simulink model "path_following_PID_v2"  (R2022a)
settings: Solver=VariableStepAuto  StartTime=0.0  StopTime=10  RelTol=1e-3
values from neighbouring files (symbols this model uses):
  ref = [x_ref, y_ref]    [reference.m]
libraries: slpidlib x1
settings Model: Creator=andreagottardini  LastModifiedBy=andreagottardini

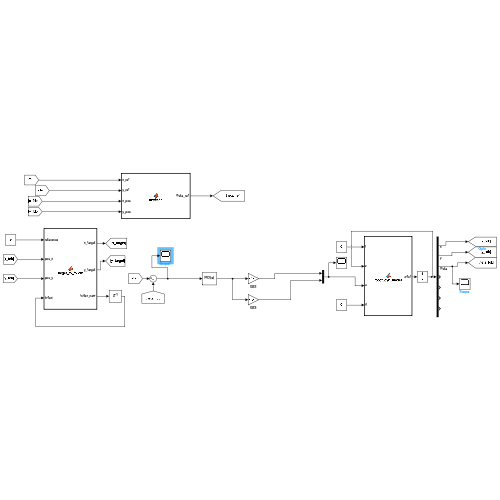
[thumbnail: Simulink's stored preview of the top-level diagram]
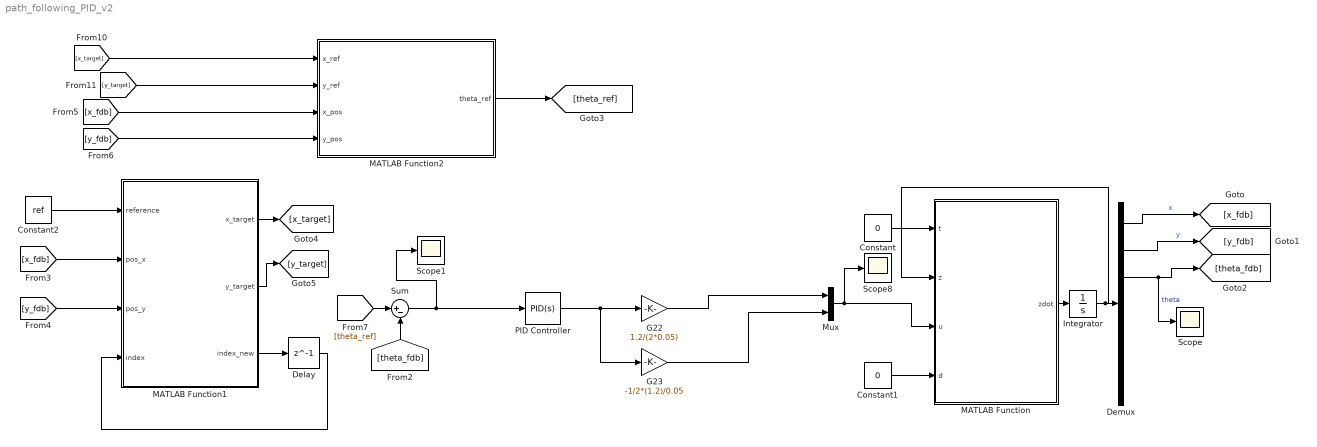
== system path_following_PID_v2 ==
  Constant : Constant  Value=0
  Constant1 : Constant  Value=0
  Constant2 : Constant  Value=ref
  Delay : Delay  DelayLength=1  InitialCondition=1
  Demux : Demux  Outputs=7
  G22 : Gain  Gain=1.2/(2*0.05)
  G23 : Gain  Gain=-1/2*(1.2)/0.05
  Integrator : Integrator  InitialCondition=[0;0;0;0;0;0;0]
  MATLAB Function : MATLAB Function  TreatAsAtomicUnit=on
  MATLAB Function1 : MATLAB Function  TreatAsAtomicUnit=on
  MATLAB Function2 : MATLAB Function  TreatAsAtomicUnit=on
  Mux : Mux  Inputs=2
  PID Controller : slpidlib/PID Controller  Controller=PID  Form=Parallel  TimeDomain=Continuous-time  UseExternalTs=off  SampleTime=-1  IntegratorMethod=Forward Euler  FilterMethod=Forward Euler  ControllerParametersSource=internal  P=0  I=1  UseKiTs=off  D=0  N=30  UseFilter=on  TunerSelectOption=Transfer Function Based (PID Tuner App)  InitialConditionSource=internal  InitialConditionForIntegrator=0  InitialConditionForFilter=0  DifferentiatorICPrevScaledInput=0  ExternalReset=none  TrackingMode=off  Kt=1  LimitOutput=off  SatLimitsSource=internal  UpperSaturationLimit=inf  LowerSaturationLimit=-inf  LinearizeAsGain=on  AntiWindupMode=none  Kb=1  POutMin=[]  POutMax=[]  IOutMin=[]  IOutMax=[]  DOutMin=[]  DOutMax=[]  NOutMin=[]  NOutMax=[]  SumOutMin=[]  SumOutMax=[]  SaturationOutMin=[]  SaturationOutMax=[]  PParamMin=[]  PParamMax=[]  IParamMin=[]  IParamMax=[]  DParamMin=[]  DParamMax=[]  NParamMin=[]  NParamMax=[]  KbParamMin=[]  KbParamMax=[]  KtParamMin=[]  KtParamMax=[]  KbOutMin=[]  KbOutMax=[]  KtOutMin=[]  KtOutMax=[]  IntegratorOutMin=[]  IntegratorOutMax=[]  FilterOutMin=[]  FilterOutMax=[]  SumI1OutMin=[]  SumI1OutMax=[]  SumI2OutMin=[]  SumI2OutMax=[]  SumI3OutMin=[]  SumI3OutMax=[]  SumI4OutMin=[]  SumI4OutMax=[]  SumDOutMin=[]  SumDOutMax=[]  DifferentiatorOutMin=[]  DifferentiatorOutMax=[]  FilterDiffOutCoefMin=[]  FilterDiffOutCoefMax=[]  ReciprocalOutMin=[]  ReciprocalOutMax=[]  SumDenOutMin=[]  SumDenOutMax=[]  SumNumOutMin=[]  SumNumOutMax=[]  DivideOutMin=[]  DivideOutMax=[]  UdiffTsProdOutMin=[]  UdiffTsProdOutMax=[]  NTsProdOutMin=[]  NTsProdOutMax=[]  UintegralTsProdOutMin=[]  UintegralTsProdOutMax=[]  UngainTsProdOutMin=[]  UngainTsProdOutMax=[]  IntegratorContinuousStateAttributes=''  IntegratorStateMustResolveToSignalObject=off  IntegratorRTWStateStorageClass=Auto  FilterContinuousStateAttributes=''  FilterStateMustResolveToSignalObject=off  FilterRTWStateStorageClass=Auto  ParallelPVariant=InternalParameters  IdealPVariant=Disabled  IVariant=InternalParameters  DVariant=InternalParameters  IntegratorVariant=Continuous  SatVariant=Disabled  AWVariant=Passthrough  PCopyVariant=Disabled  TRVariant=Disabled  FdbkBlocksVariant=Forward  IdealPFdbkVariant=Disabled  SatFdbkVariant=Disabled  DerivativeFilterVariant=ContFilter  NVariant=InternalParameters  NCopyVariant=Disabled  FilterICVariant=InternalICsFilter  IntegratorICVariant=InternalICs  ExternalResetVariant=Disabled  TRSumVariant=Passthrough  SumFdbkVariant=Disabled  SumVariant=Sum_PID  TsampFilterVariant=InternalTs  TsampNgainVariant=Passthrough  TsampIntegralVariant=Passthrough  ExternalSaturationOutDataTypeStr=Inherit: Same as second input  aMode=0
  Scope : Scope
  Scope1 : Scope
  Scope8 : Scope
  Sum : Sum  Inputs=|+-
  wires:
  Constant/1 -> MATLAB Function/1(t)
  Constant1/1 -> MATLAB Function/4(d)
  Mux/1 -> Scope8/1, MATLAB Function/3(u)
  Integrator/1 -> MATLAB Function/2(z), Demux/1
  MATLAB Function/1(zdot) -> Integrator/1
  PID Controller/1 -> G22/1, G23/1
  Sum/1 -> Scope1/1, PID Controller/1
  Demux/1 -> [x_fdb]  "x"
  Demux/2 -> [y_fdb]  "y"
  Demux/3 -> Scope/1, [theta_fdb]  "theta"
  [theta_fdb] -> Sum/2
  MATLAB Function1/1(x_target) -> [x_target]
  MATLAB Function1/3(index_new) -> Delay/1
  Delay/1 -> MATLAB Function1/4(index)
  Constant2/1 -> MATLAB Function1/1(reference)
  [x_fdb] -> MATLAB Function1/2(pos_x)
  [y_fdb] -> MATLAB Function1/3(pos_y)
  [x_fdb] -> MATLAB Function2/3(x_pos)
  [y_fdb] -> MATLAB Function2/4(y_pos)
  MATLAB Function2/1(theta_ref) -> [theta_ref]
  [theta_ref] -> Sum/1
  MATLAB Function1/2(y_target) -> [y_target]
  [x_target] -> MATLAB Function2/1(x_ref)
  [y_target] -> MATLAB Function2/2(y_ref)
  G22/1 -> Mux/1
  G23/1 -> Mux/2

== matlab function path_following_PID_v2/MATLAB Function1 ==
  data: reference input; x_target output; pos_x input; pos_y input; index input; y_target output; index_new output
function [x_target, y_target, index_new] = target_to_follow(reference, pos_x, pos_y, index)

current_target_x = reference(index,1);
current_target_y = reference(index,2);

distance = sqrt((current_target_x - pos_x)^2+(current_target_y - pos_y)^2);

if distance <= 1
    index_new = index + 1;
else
    index_new = index;
end


x_target = reference(index_new,1);
y_target = reference(index_new,2);


end

== matlab function path_following_PID_v2/MATLAB Function ==
  data: t input; z input; u input; zdot output; d input
function zdot=robot_dyn_model(t,z,u,d)

%% Read parameters, states and inputs

% Parameters
% Ic      =       th(1,1);     %
% Iw      =       th(2,1);     % 
% d       =       th(3,1);     % 
% mw      =       th(4,1);     % 
% mc      =       th(5,1);     % 
% Im      =       th(6,1);     % 
% R       =       th(7,1);     % 
% L       =       th(8,1);     % 

 Ic      =       1;     %
 Iw      =       0.1;     % 
 d       =       0.05;     % 
 mw      =       0.1;     % 
 mc      =       1;     % 
 Im      =       0.1;     % 
 R       =       0.025;     % 
 L       =       0.05;

mT = mc+2*mw;
I = Ic+mc*d^2+2*mw*L^2+2*Im;


% States
xa                  =       z(1,1);    % inertial X position (m)
ya                  =       z(2,1);    % inertial Y position (m)
theta               =       z(3,1);    % body orientation - yaw angle(rad)
phir                =       z(4,1);    % angular displacement right wheel (rad)
phil                =       z(5,1);    % angular displacement left wheel (rad)
phir_dot            =       z(6,1);    % angular velocity right wheel (rad/s)    
phil_dot            =       z(7,1);    % angular velocity left wheel (rad/s)



% Additional paramaeters
cth = cos(theta);
sth = sin(theta);

lam = [-sth     cth     0;
        cth     sth     L;
        cth     sth     -L];

b = inv(lam)*[0; R*phir_dot; R*phil_dot];

xa_dot      =    b(1,1);
ya_dot      =    b(2,1);
theta_dot   =    b(3,1);




% Inputs
taur      =       u(1,1);     % driving/braking torque right wheel (N*m)
taul      =       u(2,1);     % driving/braking torque left wheel (N*m)


%% Matrices


S = [R/(2*L)*(L*cth-d*sth) R/(2*L)*(L*cth+d*sth);
     R/(2*L)*(L*sth+d*cth) R/(2*L)*(L*sth-d*cth);
     R/(2*L)               -R/(2*L)             ;
     1                      0                   ;
     0                      1];


M_bar = [Iw+R^2/(4*L^2)*(mT*L^2+I)          R^2/(4*L^2)*(mT*L^2-I); 
        R^2/(4*L^2)*(mT*L^2-I)              Iw+R^2/(4*L^2)*(mT*L^2+I)];

V_bar = [0                              R^2/(2*L)*mc*d*theta_dot;
        -R^2/(2*L)*mc*d*theta_dot               0];



% Model equations

zdot = zeros(7,1);

zdot = [S*z(6:7,1); zeros(2,1)] + [zeros(5,2); eye(2)]*inv(M_bar)*(u-V_bar*z(6:7,1));

== matlab function path_following_PID_v2/MATLAB Function2 ==
  data: x_ref input; theta_ref output; y_ref input; x_pos input; y_pos input
function theta_ref = direction (x_ref, y_ref, x_pos, y_pos)

if (x_ref >= x_pos && y_ref >= y_pos)
    theta_ref = atan((y_ref-y_pos)/(x_ref-x_pos));
elseif (x_ref <= x_pos && y_ref >= y_pos)
    theta_ref = atan((y_ref-y_pos)/(x_pos-x_ref)) + pi/2;
elseif (x_ref <= x_pos && y_ref <= y_pos)
    theta_ref = atan((y_pos-y_ref)/(x_pos-x_ref)) + pi;
else 
    theta_ref = atan((x_ref-x_pos)/(y_pos-y_ref)) - pi/2;
end

end
